simulink model "PVModel_MT_111118"  (R2018a)
settings: Solver=FixedStepDiscrete  StartTime=0.0  StopTime=1  RelTol=1e-3
undefined symbols (not defined in the file): sigbuilder_block
libraries: powerlib x39, powerlib_meascontrol x3, simulink x2, re_lib x1
settings Model: Creator=jasil  LastModifiedBy=Michael
settings SFSimCC: SimUseLocalCustomCode=on
settings RTWCC: RTWUseLocalCustomCode=on
settings CodeAppCC: StateflowObjectComments=on

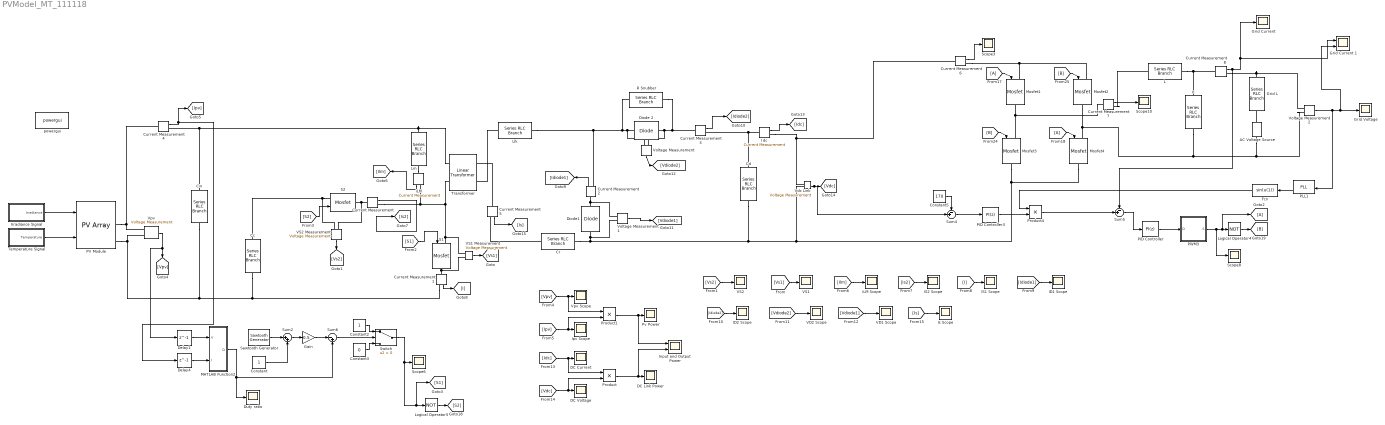
== system PVModel_MT_111118 ==
  AC Voltage Source : powerlib/Electrical Sources/AC Voltage Source  Amplitude=120*sqrt(2)  Phase=0  Frequency=60  SampleTime=0  Measurements=None  BusType=swing  Pref=10e3  Qref=0  Qmin=-inf  Qmax=+inf
      settings: SourceProductName=Simscape Electrical
  C : powerlib/Elements/Series RLC Branch  LConnTagsString=__new0  RConnTagsString=__new0  BranchType=RC  Resistance=70e-3  Inductance=1e-3  SetiL0=off  InitialCurrent=0  Capacitance=10e-6  Setx0=off  InitialVoltage=0  Measurements=None
      settings: SourceProductName=Simscape Electrical
  Cc : powerlib/Elements/Series RLC Branch  LConnTagsString=__new0  RConnTagsString=__new0  BranchType=RC  Resistance=0.000001  Inductance=1e-3  SetiL0=off  InitialCurrent=0  Capacitance=4e-6  Setx0=off  InitialVoltage=0  Measurements=None
      settings: SourceProductName=Simscape Electrical
  Cd : powerlib/Elements/Series RLC Branch  LConnTagsString=__new0  RConnTagsString=__new0  BranchType=RC  Resistance=0.000001  Inductance=1e-3  SetiL0=off  InitialCurrent=0  Capacitance=1e-3  Setx0=off  InitialVoltage=0  Measurements=None
      settings: SourceProductName=Simscape Electrical
  Cin : powerlib/Elements/Series RLC Branch  LConnTagsString=__new0  RConnTagsString=__new0  BranchType=RC  Resistance=0.000001  Inductance=1e-3  SetiL0=off  InitialCurrent=0  Capacitance=1e-3  Setx0=off  InitialVoltage=0  Measurements=Branch voltage
      settings: SourceProductName=Simscape Electrical
  Constant : Constant
  Constant2 : Constant
  Constant3 : Constant  Value=0
  Constant5 : Constant  Value=170
  Cr : powerlib/Elements/Series RLC Branch  LConnTagsString=__new0  RConnTagsString=__new0  BranchType=RC  Resistance=0.000001  Inductance=1e-3  SetiL0=off  InitialCurrent=0  Capacitance=2e-6  Setx0=off  InitialVoltage=0  Measurements=None
      settings: SourceProductName=Simscape Electrical
  Current Measurement{,1..8} (9 alike) : powerlib/Measurements/Current Measurement  PhasorSimulation=off  OutputType=Complex  PSBequivalent=0
      settings: SourceProductName=Simscape Electrical
  DC Current : Scope
  DC Link Power : Scope
  DC Voltage : Scope
  Delay1 : Delay  DelayLength=1  InitialCondition=0  SampleTime=0.01
  Delay4 : Delay  DelayLength=1  InitialCondition=0  SampleTime=.01
  Diode 2 : powerlib/Power Electronics/Diode  Ron=1  Lon=0  Vf=0.8  IC=0  UseSnubber=0  Rs=inf  Cs=0  Measurements=off
      settings: SourceProductName=Simscape Electrical
  Diode1 : powerlib/Power Electronics/Diode  Ron=0.01  Lon=0  Vf=0.8  IC=0  UseSnubber=0  Rs=inf  Cs=0  Measurements=off
      settings: SourceProductName=Simscape Electrical
  Duty ratio : Scope
  Fcn : Fcn  Expr=sin(u(1))
  Gain : Gain  Gain=0.5
  "Grid Current " : Scope
  Grid Current 1 : Scope  NumInputPorts=2
  Grid L : powerlib/Elements/Series RLC Branch  LConnTagsString=__new0  RConnTagsString=__new0  BranchType=RL  Resistance=10e-3  Inductance=2e-6  SetiL0=off  InitialCurrent=0  Capacitance=1e-6  Setx0=off  InitialVoltage=0  Measurements=None
      settings: SourceProductName=Simscape Electrical
  Grid Voltage : Scope
  I dc : powerlib/Measurements/Current Measurement  PhasorSimulation=off  OutputType=Complex  PSBequivalent=0
      settings: SourceProductName=Simscape Electrical
  ID1 Scope : Scope
  ID2 Scope : Scope
  IS1 Scope : Scope
  IS2 Scope : Scope
  Input and Output Power : Scope  NumInputPorts=2
  Ipv Scope : Scope
  "Irradiance Signal " : Subsystem  Tag=STV Subsys  LoadFcn=sigbuilder_block('load');  StartFcn=sigbuilder_block('start');  StopFcn=sigbuilder_block('stop');  ClipboardFcn=sigbuilder_block('clipboard');  mask(Sigbuilder block){tuvar=[0:10]}
      mask help: Simulink:masks:SigbuilderBlock_MD
      mask init:
      | if ~strcmp(get_param(bdroot(gcbh),'SimulationStatus'),'stopped') tuvar = sigbuilder_block('maskInit'); end
      settings: CopyFcn=sigbuilder_block('copy');  DeleteFcn=sigbuilder_block('delete');  ModelCloseFcn=sigbuilder_block('modelClose');  PreSaveFcn=sigbuilder_block('preSave');  PauseFcn=sigbuilder_block('pause');  ContinueFcn=sigbuilder_block('continue');  NameChangeFcn=sigbuilder_block('namechange');  OpenFcn=sigbuilder_block('open',[6 30 1012.5 447.75 ]);  CloseFcn=sigbuilder_block('close');
      mask Display: plot(0, 0, 100, 100,[2, 2, 32, 32, 2], [68, 8, 8, 68, 68],[32, 2], [38, 38], [32, 19, 2],[53, 60, 44], [32, 17, 17, 2],[16, 16, 31, 31]);txt = getActiveGroup(gcbh);text(2, 100, txt,'verticalAlignment', 'top');
  Is Scope : Scope
  L : powerlib/Elements/Series RLC Branch  LConnTagsString=__new0  RConnTagsString=__new0  BranchType=RL  Resistance=70e-3  Inductance=40e-3  SetiL0=off  InitialCurrent=0  Capacitance=1e-6  Setx0=off  InitialVoltage=0  Measurements=None
      settings: SourceProductName=Simscape Electrical
  Llk : powerlib/Elements/Series RLC Branch  LConnTagsString=__new0  RConnTagsString=__new0  BranchType=RL  Resistance=0.000001  Inductance=2.6e-6  SetiL0=off  InitialCurrent=0  Capacitance=1e-6  Setx0=off  InitialVoltage=0  Measurements=None
      settings: SourceProductName=Simscape Electrical
  Lm : powerlib/Elements/Series RLC Branch  LConnTagsString=__new0  RConnTagsString=__new0  BranchType=RL  Resistance=0.000001  Inductance=10e-6  SetiL0=off  InitialCurrent=0  Capacitance=1e-6  Setx0=off  InitialVoltage=0  Measurements=None
      settings: SourceProductName=Simscape Electrical
  Logical Operator4 : Logic  Operator=NOT  AllPortsSameDT=off  OutDataTypeStr=boolean
  Logical Operator5 : Logic  Operator=NOT  AllPortsSameDT=off  OutDataTypeStr=boolean
  MATLAB Function2 : MATLAB Function  TreatAsAtomicUnit=on
  Mosfet{1..4} (4 alike) : powerlib/Power Electronics/Mosfet  Ron=0.1  Lon=0  Rd=0.01  Vfd=0  IC=0  Rs=1e5  Cs=inf  Measurements=off
      settings: SourceProductName=Simscape Electrical
  PID Controller : simulink/Continuous/PID Controller  Controller=PI  Form=Parallel  TimeDomain=Discrete-time  SampleTime=-1  IntegratorMethod=Forward Euler  FilterMethod=Forward Euler  ControllerParametersSource=internal  P=10  I=100  D=0  UseFilter=on  N=100  TunerSelectOption=Transfer Function Based (PID Tuner App)  InitialConditionSource=internal  InitialConditionForIntegrator=0  InitialConditionForFilter=0  DifferentiatorICPrevScaledInput=0  ExternalReset=none  TrackingMode=off  Kt=1  LimitOutput=off  UpperSaturationLimit=inf  LowerSaturationLimit=-inf  LinearizeAsGain=on  AntiWindupMode=none  Kb=1  POutMin=[]  POutMax=[]  IOutMin=[]  IOutMax=[]  DOutMin=[]  DOutMax=[]  NOutMin=[]  NOutMax=[]  SumOutMin=[]  SumOutMax=[]  SaturationOutMin=[]  SaturationOutMax=[]  PParamMin=[]  PParamMax=[]  IParamMin=[]  IParamMax=[]  DParamMin=[]  DParamMax=[]  NParamMin=[]  NParamMax=[]  KbParamMin=[]  KbParamMax=[]  KtParamMin=[]  KtParamMax=[]  KbOutMin=[]  KbOutMax=[]  KtOutMin=[]  KtOutMax=[]  IntegratorOutMin=[]  IntegratorOutMax=[]  FilterOutMin=[]  FilterOutMax=[]  SumI1OutMin=[]  SumI1OutMax=[]  SumI2OutMin=[]  SumI2OutMax=[]  SumI3OutMin=[]  SumI3OutMax=[]  SumDOutMin=[]  SumDOutMax=[]  DifferentiatorOutMin=[]  DifferentiatorOutMax=[]  FilterDiffOutCoefMin=[]  FilterDiffOutCoefMax=[]  ReciprocalOutMin=[]  ReciprocalOutMax=[]  SumDenOutMin=[]  SumDenOutMax=[]  SumNumOutMin=[]  SumNumOutMax=[]  DivideOutMin=[]  DivideOutMax=[]  IntegratorContinuousStateAttributes=''  IntegratorStateMustResolveToSignalObject=off  IntegratorRTWStateStorageClass=Auto  FilterContinuousStateAttributes=''  FilterStateMustResolveToSignalObject=off  FilterRTWStateStorageClass=Auto
  PID Controller3 : simulink/Continuous/PID Controller  Controller=PI  Form=Parallel  TimeDomain=Discrete-time  SampleTime=-1  IntegratorMethod=Forward Euler  FilterMethod=Forward Euler  ControllerParametersSource=internal  P=0.25  I=20  D=0  UseFilter=on  N=100  TunerSelectOption=Transfer Function Based (PID Tuner App)  InitialConditionSource=internal  InitialConditionForIntegrator=0  InitialConditionForFilter=0  DifferentiatorICPrevScaledInput=0  ExternalReset=none  TrackingMode=off  Kt=1  LimitOutput=off  UpperSaturationLimit=inf  LowerSaturationLimit=-inf  LinearizeAsGain=on  AntiWindupMode=none  Kb=1  POutMin=[]  POutMax=[]  IOutMin=[]  IOutMax=[]  DOutMin=[]  DOutMax=[]  NOutMin=[]  NOutMax=[]  SumOutMin=[]  SumOutMax=[]  SaturationOutMin=[]  SaturationOutMax=[]  PParamMin=[]  PParamMax=[]  IParamMin=[]  IParamMax=[]  DParamMin=[]  DParamMax=[]  NParamMin=[]  NParamMax=[]  KbParamMin=[]  KbParamMax=[]  KtParamMin=[]  KtParamMax=[]  KbOutMin=[]  KbOutMax=[]  KtOutMin=[]  KtOutMax=[]  IntegratorOutMin=[]  IntegratorOutMax=[]  FilterOutMin=[]  FilterOutMax=[]  SumI1OutMin=[]  SumI1OutMax=[]  SumI2OutMin=[]  SumI2OutMax=[]  SumI3OutMin=[]  SumI3OutMax=[]  SumDOutMin=[]  SumDOutMax=[]  DifferentiatorOutMin=[]  DifferentiatorOutMax=[]  FilterDiffOutCoefMin=[]  FilterDiffOutCoefMax=[]  ReciprocalOutMin=[]  ReciprocalOutMax=[]  SumDenOutMin=[]  SumDenOutMax=[]  SumNumOutMin=[]  SumNumOutMax=[]  DivideOutMin=[]  DivideOutMax=[]  IntegratorContinuousStateAttributes=''  IntegratorStateMustResolveToSignalObject=off  IntegratorRTWStateStorageClass=Auto  FilterContinuousStateAttributes=''  FilterStateMustResolveToSignalObject=off  FilterRTWStateStorageClass=Auto
  PLL1 : powerlib_meascontrol/PLL/PLL  Fmin=60  Par_Init=[0, 60]  ParK=[180, 3200, 1]  TcD=1e-4  MaxRateChangeFreq=12  FilterCutOffFreq=25  Ts=1e-6  AGC=on
      settings: SourceProductName=Simscape Electrical  SourceProductBaseCode=PS
  PV Module : re_lib/Solar/PV Array  Npar=1  Nser=1  PlotType=array @ 25 deg.C & specified irradiances  S_vec="[ 1000  500  100 ]"  Temp_C_vec="[ 45 25  ]"  ModuleName=User-defined  PlotWhenSelected=off  Pm=179.9805  Ncell=36  Voc=24.06  Isc=9.77  Vm=19.67  Im=9.15  beta_Voc_pc=-0.28  alpha_Isc_pc=+0.04  beta_Voc=-0.067368  alpha_Isc=0.003908  IL=9.8911  I0=1.3829e-11  nI=0.95443  Rsh=60.4787  Rs=0.18212  BAL=off  Tc=1e-6  Tfilter=5e-5
      settings: SourceProductName=Simscape Electrical
  PWM3 : Subsystem
  Product : Product
  Product1 : Product
  Product4 : Product
  Pv Power : Scope
  R Snubber : powerlib/Elements/Series RLC Branch  LConnTagsString=__new0  RConnTagsString=__new0  BranchType=R  Resistance=1e6  Inductance=1e-3  SetiL0=off  InitialCurrent=0  Capacitance=1e-6  Setx0=off  InitialVoltage=0  Measurements=None
      settings: SourceProductName=Simscape Electrical
  S1 : powerlib/Power Electronics/Mosfet  Ron=5.6e-3  Lon=0  Rd=0.01  Vfd=1.3  IC=0  Rs=1e6  Cs=inf  Measurements=off
      settings: SourceProductName=Simscape Electrical
  S2 : powerlib/Power Electronics/Mosfet  Ron=5.6e-3  Lon=0  Rd=0.01  Vfd=1.3  IC=0  Rs=1e5  Cs=inf  Measurements=off
      settings: SourceProductName=Simscape Electrical
  Sawtooth Generator : powerlib_meascontrol/Pulse & Signal Generators/Sawtooth Generator  Freq=50000  Phase=180  Ts=0
      settings: SourceProductName=Simscape Electrical
  Scope{3,6,8,10} (4 alike) : Scope
  Sum2 : Sum  Inputs=|++
  Sum4 : Sum  Inputs=-+|
  Sum5 : Sum  Inputs=-+|
  Sum6 : Sum  Inputs=|-+
  Switch : Switch  Criteria=u2 > Threshold
  Temperature Signal : Subsystem  Tag=STV Subsys  LoadFcn=sigbuilder_block('load');  StartFcn=sigbuilder_block('start');  StopFcn=sigbuilder_block('stop');  ClipboardFcn=sigbuilder_block('clipboard');  mask(Sigbuilder block){tuvar=[0:10]}
      mask help: Simulink:masks:SigbuilderBlock_MD
      mask init:
      | if ~strcmp(get_param(bdroot(gcbh),'SimulationStatus'),'stopped') tuvar = sigbuilder_block('maskInit'); end
      settings: CopyFcn=sigbuilder_block('copy');  DeleteFcn=sigbuilder_block('delete');  ModelCloseFcn=sigbuilder_block('modelClose');  PreSaveFcn=sigbuilder_block('preSave');  PauseFcn=sigbuilder_block('pause');  ContinueFcn=sigbuilder_block('continue');  NameChangeFcn=sigbuilder_block('namechange');  OpenFcn=sigbuilder_block('open',[6 30 1012.5 447.75 ]);  CloseFcn=sigbuilder_block('close');
      mask Display: plot(0, 0, 100, 100,[2, 2, 32, 32, 2], [68, 8, 8, 68, 68],[32, 2], [38, 38], [32, 19, 2],[53, 60, 44], [32, 17, 17, 2],[16, 16, 31, 31]);txt = getActiveGroup(gcbh);text(2, 100, txt,'verticalAlignment', 'top');
  Transformer : powerlib/Elements/Linear Transformer  UNITS=SI  NominalPower=[ 25 100e3 ]  winding1=[6.36 0 0]  winding2=[26.87 0 0]  ThreeWindings=off  winding3=[3.15e+05 3.969e+07 6316.9]  RmLm=[1e6 Inf]  Measurements=None  DataType=on
      settings: SourceProductName=Simscape Electrical
  VD1 Scope : Scope
  VD2 Scope : Scope
  VS1 : Scope
  VS1 Measurement : powerlib/Measurements/Voltage Measurement  PhasorSimulation=off  OutputType=Complex  PSBequivalent=0
      settings: SourceProductName=Simscape Electrical
  VS2 : Scope
  VS2 Measurement : powerlib/Measurements/Voltage Measurement  PhasorSimulation=off  OutputType=Complex  PSBequivalent=0
      settings: SourceProductName=Simscape Electrical
  Vdc Link : powerlib/Measurements/Voltage Measurement  PhasorSimulation=off  OutputType=Complex  PSBequivalent=0
      settings: SourceProductName=Simscape Electrical
  Voltage Measurement : powerlib/Measurements/Voltage Measurement  PhasorSimulation=off  OutputType=Complex  PSBequivalent=0
      settings: SourceProductName=Simscape Electrical
  Voltage Measurement1 : powerlib/Measurements/Voltage Measurement  PhasorSimulation=off  OutputType=Complex  PSBequivalent=0
      settings: SourceProductName=Simscape Electrical
  Voltage Measurement2 : powerlib/Measurements/Voltage Measurement  PhasorSimulation=off  OutputType=Complex  PSBequivalent=0
      settings: SourceProductName=Simscape Electrical
  Vpv : powerlib/Measurements/Voltage Measurement  PhasorSimulation=off  OutputType=Complex  PSBequivalent=0
      settings: SourceProductName=Simscape Electrical
  Vpv Scope : Scope
  iLM : powerlib/Measurements/Current Measurement  PhasorSimulation=off  OutputType=Complex  PSBequivalent=0
      settings: SourceProductName=Simscape Electrical
  iLM Scope : Scope
  powergui : powerlib/powergui  Priority=1  SimulationMode=Discrete  SampleTime=1e-7  frequency=60  Iterations=50  frequencyindice=0  Pbase=100e6  ErrMax=1e-4  UnitsV=kV  UnitsW=MW  buscounter=0  FunctionMessages=off  echomessages=off  EnableUseOfTLC=off  CurrentSourceSwitches=off  DisableSnubberDevices=off  DisableRonSwitches=off  DisableVfSwitches=off  DisplayEquations=off  SolverType=Tustin/Backward Euler (TBE)  Interpol=off  ExternalGateDelay=off  methode=off  Ts=100  x0status=blocks  SPID=on  SwTol=0  HookPort=off  RestoreLinks=warning  ResistiveCurrentMeasurement=off  Frange=[0:2:500]  Ylog=off  Xlog=on  ShowGrid=off  save=off  variable=ZData  structure=0  ZoomFFT=off  StartTime=0.0  cycles=1  DisplayStyle=1  fundamental=60  FreqAxis=off  MaxFrequency=1000  frequencyindicesteady=1  RmsSteady=1  display=off
  wires:
  [Vdiode1] -> VD1 Scope/1
  "Irradiance Signal "/1(Irradiance) -> PV Module/1
  [Vdc] -> Product/2, DC Voltage/1
  VS2 Measurement/1 -> [Vs2]
  Current Measurement1/1 -> [I]
  Vpv/1 -> Delay1/1, [Vpv]
  Voltage Measurement/1 -> [Vdiode2]
  Voltage Measurement1/1 -> [Vdiode1]
  [S2] -> S2/1
  Current Measurement2/1 -> [Idiode1]
  [Vdiode2] -> VD2 Scope/1
  [Idiode1] -> ID1 Scope/1
  [Vpv] -> Product1/1, Vpv Scope/1
  [Ipv] -> Product1/2, Ipv Scope/1
  Current Measurement/1 -> [Is2]
  [Vs1] -> VS1/1
  [S1] -> S1/1
  [I] -> IS1 Scope/1
  [Vs2] -> VS2/1
  iLM/1 -> [Ilm]
  Product/1 -> Input and Output Power/2, DC Link Power/1
  [Ilm] -> iLM Scope/1
  [Idiode2] -> ID2 Scope/1
  Product1/1 -> Input and Output Power/1, Pv Power/1
  [Is2] -> IS2 Scope/1
  VS1 Measurement/1 -> [Vs1]
  [Idc] -> Product/1, DC Current/1
  Temperature Signal/1(Temperature) -> PV Module/2
  [Is] -> Is Scope/1
  Current Measurement4/1 -> Delay4/1, [Ipv]
  I dc/1 -> [Idc]
  Current Measurement3/1 -> [Idiode2]
  Current Measurement5/1 -> [Is]
  [A] -> Mosfet4/1
  PID Controller3/1 -> Product4/2
  Product4/1 -> Sum5/2
  Constant5/1 -> Sum4/1
  Voltage Measurement2/1 -> Grid Current 1/2, Grid Voltage/1, PLL1/1
  Current Measurement8/1 -> Grid Current 1/1, "Grid Current "/1, Sum5/1
  PLL1/2 -> Fcn/1
  [A] -> Mosfet1/1
  Current Measurement7/1 -> Scope10/1
  Logical Operator4/1 -> [B]
  Vdc Link/1 -> Sum4/2, [Vdc]
  Fcn/1 -> Product4/1
  Current Measurement6/1 -> Scope3/1
  [B] -> Mosfet3/1
  PID Controller/1 -> PWM3/1(D)
  Sum4/1 -> PID Controller3/1
  PWM3/1(S) -> Scope8/1, [A], Logical Operator4/1
  Sum5/1 -> PID Controller/1
  [B] -> Mosfet2/1
  Delay4/1 -> MATLAB Function2/2(I)
  MATLAB Function2/1(D) -> Sum6/2, Duty ratio/1
  Sum6/1 -> Switch/2
  Constant2/1 -> Switch/1
  Delay1/1 -> MATLAB Function2/1(V)
  Sum2/1 -> Gain/1
  Constant/1 -> Sum2/2
  Constant3/1 -> Switch/3
  Sawtooth Generator/1 -> Sum2/1
  Gain/1 -> Sum6/1
  Switch/1 -> [S1], Logical Operator5/1, Scope6/1
  Logical Operator5/1 -> [S2]
  connections:
  Current Measurement1/RConn1 -- Vpv/LConn2 -- PV Module/RConn2 -- Cin/RConn1 -- Cc/RConn1
  Llk/RConn1 -- R Snubber/LConn1 -- Voltage Measurement/LConn2 -- Diode 2/LConn1 -- Current Measurement2/RConn1
  VS1 Measurement/LConn2 -- Current Measurement1/LConn1 -- S1/RConn1
  S2/LConn1 -- VS2 Measurement/LConn1 -- Cc/LConn1
  iLM/RConn1 -- S1/LConn1 -- VS1 Measurement/LConn1 -- Transformer/LConn2 -- Current Measurement/RConn1
  Cd/LConn1 -- I dc/LConn1 -- Current Measurement3/RConn1
  S2/RConn1 -- VS2 Measurement/LConn2 -- Current Measurement/LConn1
  Lm/RConn1 -- iLM/LConn1
  Cr/LConn1 -- Current Measurement5/RConn1
  I dc/RConn1 -- Current Measurement6/LConn1 -- Vdc Link/LConn1
  Lm/LConn1 -- Cin/LConn1 -- Current Measurement4/RConn1 -- Transformer/LConn1
  PV Module/RConn1 -- Vpv/LConn1 -- Current Measurement4/LConn1
  Diode 2/RConn1 -- Voltage Measurement/LConn1 -- R Snubber/RConn1 -- Current Measurement3/LConn1
  Diode1/RConn1 -- Voltage Measurement1/LConn1 -- Current Measurement2/LConn1
  Mosfet4/RConn1 -- Vdc Link/LConn2 -- Cr/RConn1 -- Voltage Measurement1/LConn2 -- Diode1/LConn1 -- Cd/RConn1 -- Mosfet3/RConn1
  Current Measurement8/RConn1 -- Grid L/LConn1 -- Voltage Measurement2/LConn1
  Mosfet4/LConn1 -- Mosfet2/RConn1 -- C/RConn1 -- Voltage Measurement2/LConn2 -- AC Voltage Source/LConn1
  Current Measurement7/LConn1 -- Mosfet1/RConn1 -- Mosfet3/LConn1
  Current Measurement6/RConn1 -- Mosfet1/LConn1 -- Mosfet2/LConn1
  L/RConn1 -- C/LConn1 -- Current Measurement8/LConn1
  AC Voltage Source/RConn1 -- Grid L/RConn1
  Current Measurement7/RConn1 -- L/LConn1
  Llk/LConn1 -- Transformer/RConn2
  Current Measurement5/LConn1 -- Transformer/RConn1

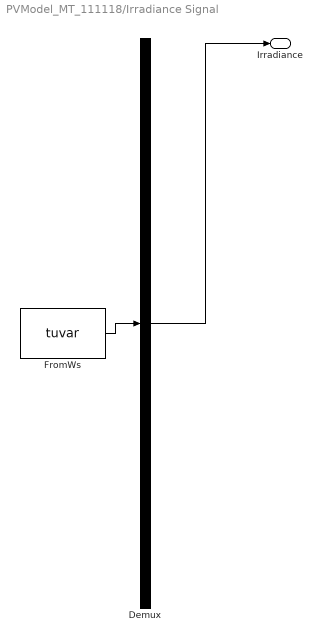
== system PVModel_MT_111118/Irradiance Signal  ==
  Demux : Demux  Tag=STV Demux  Outputs=1
  FromWs : FromWorkspace  Tag=STV FromWs  VariableName=tuvar  SampleTime=0
      SigBuilderData=|
      | common.afterFinalStr = 'Extrapolate'
      | common.sampleTime = 0
      | dataSet.timeRange = [0 0.3]
      | dataSet.name = 'Group 1'
      | sbobj.Groups.Name = 'Group 1'
      | sbobj.Groups.Signals.Name = 'Irradiance'
      | sbobj.Groups.Signals.XData = [0 0.1 0.2 0.3]
      | sbobj.Groups.Signals.YData = [1000 1000 1000 1000]
      | sbobj.Groups.TimeRange = [0 0.3]
  Irradiance : Outport  Tag=STV Outport
  wires:
  Demux/1 -> Irradiance/1
  FromWs/1 -> Demux/1

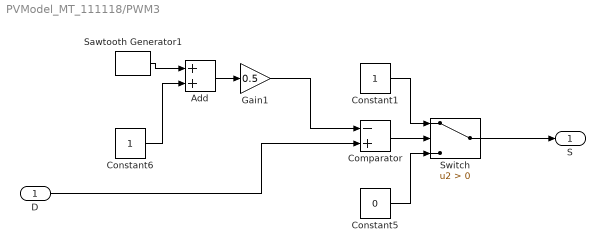
== system PVModel_MT_111118/PWM3 ==
  D : Inport
  Add : Sum
  Comparator : Sum  Inputs=-+
  Constant1 : Constant
  Constant5 : Constant  Value=0
  Constant6 : Constant
  Gain1 : Gain  Gain=0.5
  Sawtooth Generator1 : powerlib_meascontrol/Pulse & Signal Generators/Sawtooth Generator  Freq=16000  Phase=180  Ts=0
      settings: SourceProductName=Simscape Electrical
  Switch : Switch  Criteria=u2 > Threshold
  S : Outport
  wires:
  Switch/1 -> S/1
  Constant1/1 -> Switch/1
  Comparator/1 -> Switch/2
  Constant6/1 -> Add/2
  Gain1/1 -> Comparator/1
  Constant5/1 -> Switch/3
  Sawtooth Generator1/1 -> Add/1
  Add/1 -> Gain1/1
  D/1 -> Comparator/2

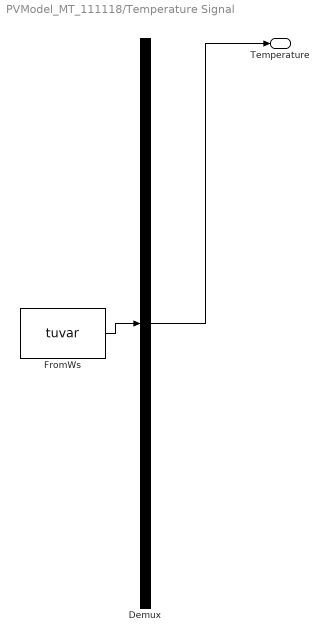
== system PVModel_MT_111118/Temperature Signal ==
  Demux : Demux  Tag=STV Demux  Outputs=1
  FromWs : FromWorkspace  Tag=STV FromWs  VariableName=tuvar  SampleTime=0
      SigBuilderData=|
      | common.afterFinalStr = 'Extrapolate'
      | common.sampleTime = 0
      | dataSet.timeRange = [0 0.3]
      | dataSet.name = 'Group 1'
      | sbobj.Groups.Name = 'Group 1'
      | sbobj.Groups.Signals.Name = 'Temperature'
      | sbobj.Groups.Signals.XData = [0 0.1 0.2 0.3]
      | sbobj.Groups.Signals.YData = [25 25 25 25]
      | sbobj.Groups.TimeRange = [0 0.3]
  Temperature : Outport  Tag=STV Outport
  wires:
  Demux/1 -> Temperature/1
  FromWs/1 -> Demux/1

== matlab function PVModel_MT_111118/MATLAB Function2 ==
  data: V input; D output; I input
function D = fcn(V,I)

persistent Dprev Pprev Vprev

% Initialize the internal values for the voltage and power on the
% first pass
if isempty(Dprev)
    Dprev = 0.54;
    Vprev = 60;
    Pprev = 500;
end

% Initialize algorithm parameters
deltaD = 0.01;

% Calculate measured array power
P = V*I;

% Increase or decrease duty cycle based on conditions
if (P-Pprev) ~= 0
    if (P-Pprev) > 0
        if (V-Vprev) > 0
            D = Dprev - deltaD;
        else
            D = Dprev + deltaD;
        end
    else
        if (V-Vprev) > 0
            D = Dprev + deltaD;
        else
            D = Dprev - deltaD;
        end        
    end
else
    D = Dprev;
end

% Update internal values
Dprev = D;
Vprev = V;
Pprev = P;

end
